simulink model "Split2"  (R2023b)
settings: Solver=VariableStepAuto  StartTime=0.0  StopTime=10.0  RelTol=1e-3
settings Model: Creator=iceki  LastModifiedBy=iceki

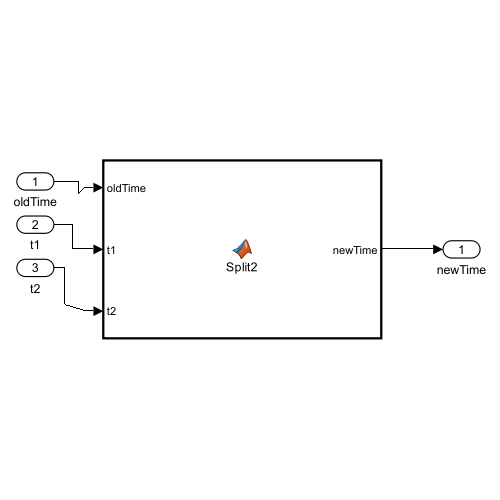
[thumbnail: Simulink's stored preview of the top-level diagram]
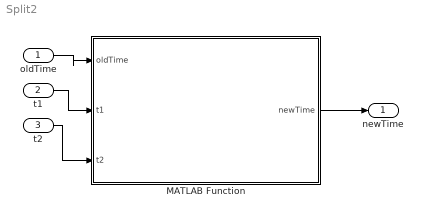
== system Split2 ==
  oldTime : Inport
  t1 : Inport  Port=2
  t2 : Inport  Port=3
  MATLAB Function : MATLAB Function  TreatAsAtomicUnit=on
  newTime : Outport
  wires:
  oldTime/1 -> MATLAB Function/1(oldTime)
  t1/1 -> MATLAB Function/2(t1)
  t2/1 -> MATLAB Function/3(t2)
  MATLAB Function/1(newTime) -> newTime/1

== matlab function Split2/MATLAB Function ==
  data: oldTime input; newTime output; t1 input; t2 input
function newTime  = Split2(oldTime,t1,t2)

M = [t1 t2];
newTime = oldTime + min(M);
end
